simulink model "Wind_turbin."  (R2022b)
settings: Solver=ode45  StartTime=0.0  StopTime=Tsim  FixedStep=5e-5  RelTol=1e-6  EnableMultiTasking=on
values from neighbouring files (symbols this model uses):
  c1 = 0.44    [wind_code.m]
  c2 = 125    [wind_code.m]
  c3 = 0    [wind_code.m]
  c4 = 0    [wind_code.m]
  c5 = 0    [wind_code.m]
  c6 = 6.94    [wind_code.m]
  c7 = 16.5    [wind_code.m]
  c8 = 0    [wind_code.m]
  c9 = -0.002    [wind_code.m]
  N = 80    [wind_code.m]
  p = 2    [wind_code.m]
undefined symbols (not defined in the file or in its folder): A, Cdc, f_n1, fluxm, Jtot, Kcp, ki_dc, ki_m, ki_P_n1, ki_pll_n1, ki_s_n1, kp_dc, kp_md, kp_mq, kp_P_n1, kp_pll_n1, kp_s_n1, Lc_n1, Ld, Lg_n1, Lq, magnitud_delay, pitch, Q_set, Rc_n1, Rg_n1, rho, Rs, Rt, t_step_Q, Vdcref_n1, Vpeak_n1, w_n1
libraries: spsControlledVoltageSourceLib x9, slpidlib x8, spsSeriesRLCBranchLib x7, spsCurrentMeasurementLib x3, spsGroundLib x2, spsThreePhaseVIMeasurementLib x2, spsControlledCurrentSourceLib x2, spsPower3phInstantaneousLib x2, spsPermanentMagnetSynchronousMachineLib x1, spsVoltageMeasurementLib x1, sps_lib x1
(part 2 of 2)

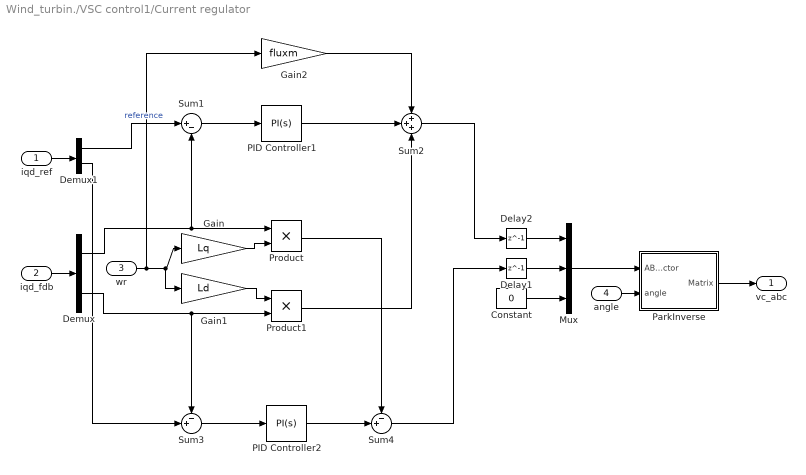
== system Wind_turbin./VSC control1/Current regulator ==
  iqd_ref : Inport
  iqd_fdb : Inport  Port=2
  wr : Inport  Port=3
  angle : Inport  Port=4
  Constant : Constant  Value=0
  Delay1 : Delay  DelayLength=1  InitialCondition=0  SampleTime=magnitud_delay
  Delay2 : Delay  DelayLength=1  InitialCondition=Vpeak_n1  SampleTime=magnitud_delay
  Demux : Demux  Outputs=2
  Demux1 : Demux  Outputs=2
  Gain : Gain  Gain=Lq
  Gain1 : Gain  Gain=Ld
  Gain2 : Gain  Gain=fluxm
  Mux : Mux  Inputs=3
  PID Controller1 : slpidlib/PID Controller  Controller=PI  Form=Parallel  TimeDomain=Continuous-time  UseExternalTs=off  SampleTime=-1  IntegratorMethod=Forward Euler  FilterMethod=Forward Euler  ControllerParametersSource=internal  P=kp_mq  I=ki_m  UseKiTs=off  D=0  N=100  UseFilter=on  TunerSelectOption=Transfer Function Based (PID Tuner App)  InitialConditionSource=internal  InitialConditionForIntegrator=0  InitialConditionForFilter=0  DifferentiatorICPrevScaledInput=0  ExternalReset=none  TrackingMode=off  Kt=1  LimitOutput=off  SatLimitsSource=internal  UpperSaturationLimit=inf  LowerSaturationLimit=-inf  LinearizeAsGain=on  AntiWindupMode=none  Kb=1  LimitIntegrator=off  UpperIntegratorSaturationLimit=inf  LowerIntegratorSaturationLimit=-inf  POutMin=[]  POutMax=[]  IOutMin=[]  IOutMax=[]  DOutMin=[]  DOutMax=[]  NOutMin=[]  NOutMax=[]  SumOutMin=[]  SumOutMax=[]  SaturationOutMin=[]  SaturationOutMax=[]  PParamMin=[]  PParamMax=[]  IParamMin=[]  IParamMax=[]  DParamMin=[]  DParamMax=[]  NParamMin=[]  NParamMax=[]  KbParamMin=[]  KbParamMax=[]  KtParamMin=[]  KtParamMax=[]  KbOutMin=[]  KbOutMax=[]  KtOutMin=[]  KtOutMax=[]  IntegratorOutMin=[]  IntegratorOutMax=[]  FilterOutMin=[]  FilterOutMax=[]  SumI1OutMin=[]  SumI1OutMax=[]  SumI2OutMin=[]  SumI2OutMax=[]  SumI3OutMin=[]  SumI3OutMax=[]  SumI4OutMin=[]  SumI4OutMax=[]  SumDOutMin=[]  SumDOutMax=[]  DifferentiatorOutMin=[]  DifferentiatorOutMax=[]  FilterDiffOutCoefMin=[]  FilterDiffOutCoefMax=[]  ReciprocalOutMin=[]  ReciprocalOutMax=[]  SumDenOutMin=[]  SumDenOutMax=[]  SumNumOutMin=[]  SumNumOutMax=[]  DivideOutMin=[]  DivideOutMax=[]  UdiffTsProdOutMin=[]  UdiffTsProdOutMax=[]  NTsProdOutMin=[]  NTsProdOutMax=[]  UintegralTsProdOutMin=[]  UintegralTsProdOutMax=[]  UngainTsProdOutMin=[]  UngainTsProdOutMax=[]  ClampingZeroOutDataTypeStr=Inherit: Inherit via back propagation  ClampingZeroOutMin=[]  ClampingZeroOutMax=[]  FilterDenConstantOutDataTypeStr=Inherit: Inherit via back propagation  FilterDenConstantOutMin=[]  FilterDenConstantOutMax=[]  PCopyOutDataTypeStr=Inherit: Inherit via back propagation  PCopyOutMin=[]  PCopyOutMax=[]  NCopyOutDataTypeStr=Inherit: Inherit via back propagation  NCopyOutMin=[]  NCopyOutMax=[]  IntegratorContinuousStateAttributes=''  IntegratorStateMustResolveToSignalObject=off  IntegratorRTWStateStorageClass=Auto  FilterContinuousStateAttributes=''  FilterStateMustResolveToSignalObject=off  FilterRTWStateStorageClass=Auto  ParallelPVariant=InternalParameters  IdealPVariant=Disabled  IVariant=InternalParameters  DVariant=Disabled  IntegratorVariant=Continuous  SatVariant=Disabled  AWVariant=Passthrough  PCopyVariant=Disabled  TRVariant=Disabled  FdbkBlocksVariant=Forward  IdealPFdbkVariant=Disabled  SatFdbkVariant=Disabled  DerivativeFilterVariant=Disabled  NVariant=Disabled  NCopyVariant=Disabled_SignalSpec  FilterICVariant=Disabled  IntegratorICVariant=InternalICs  ExternalResetVariant=Disabled  TRSumVariant=Passthrough  SumFdbkVariant=Disabled  SumVariant=Sum_PI  TsampFilterVariant=InternalTs  TsampNgainVariant=Passthrough  TsampIntegralVariant=Passthrough  ExternalSaturationOutDataTypeStr=Inherit: Same as second input
  PID Controller2 : slpidlib/PID Controller  Controller=PI  Form=Parallel  TimeDomain=Continuous-time  UseExternalTs=off  SampleTime=-1  IntegratorMethod=Forward Euler  FilterMethod=Forward Euler  ControllerParametersSource=internal  P=kp_md  I=ki_m  UseKiTs=off  D=0  N=100  UseFilter=on  TunerSelectOption=Transfer Function Based (PID Tuner App)  InitialConditionSource=internal  InitialConditionForIntegrator=0  InitialConditionForFilter=0  DifferentiatorICPrevScaledInput=0  ExternalReset=none  TrackingMode=off  Kt=1  LimitOutput=off  SatLimitsSource=internal  UpperSaturationLimit=inf  LowerSaturationLimit=-inf  LinearizeAsGain=on  AntiWindupMode=none  Kb=1  LimitIntegrator=off  UpperIntegratorSaturationLimit=inf  LowerIntegratorSaturationLimit=-inf  POutMin=[]  POutMax=[]  IOutMin=[]  IOutMax=[]  DOutMin=[]  DOutMax=[]  NOutMin=[]  NOutMax=[]  SumOutMin=[]  SumOutMax=[]  SaturationOutMin=[]  SaturationOutMax=[]  PParamMin=[]  PParamMax=[]  IParamMin=[]  IParamMax=[]  DParamMin=[]  DParamMax=[]  NParamMin=[]  NParamMax=[]  KbParamMin=[]  KbParamMax=[]  KtParamMin=[]  KtParamMax=[]  KbOutMin=[]  KbOutMax=[]  KtOutMin=[]  KtOutMax=[]  IntegratorOutMin=[]  IntegratorOutMax=[]  FilterOutMin=[]  FilterOutMax=[]  SumI1OutMin=[]  SumI1OutMax=[]  SumI2OutMin=[]  SumI2OutMax=[]  SumI3OutMin=[]  SumI3OutMax=[]  SumI4OutMin=[]  SumI4OutMax=[]  SumDOutMin=[]  SumDOutMax=[]  DifferentiatorOutMin=[]  DifferentiatorOutMax=[]  FilterDiffOutCoefMin=[]  FilterDiffOutCoefMax=[]  ReciprocalOutMin=[]  ReciprocalOutMax=[]  SumDenOutMin=[]  SumDenOutMax=[]  SumNumOutMin=[]  SumNumOutMax=[]  DivideOutMin=[]  DivideOutMax=[]  UdiffTsProdOutMin=[]  UdiffTsProdOutMax=[]  NTsProdOutMin=[]  NTsProdOutMax=[]  UintegralTsProdOutMin=[]  UintegralTsProdOutMax=[]  UngainTsProdOutMin=[]  UngainTsProdOutMax=[]  ClampingZeroOutDataTypeStr=Inherit: Inherit via back propagation  ClampingZeroOutMin=[]  ClampingZeroOutMax=[]  FilterDenConstantOutDataTypeStr=Inherit: Inherit via back propagation  FilterDenConstantOutMin=[]  FilterDenConstantOutMax=[]  PCopyOutDataTypeStr=Inherit: Inherit via back propagation  PCopyOutMin=[]  PCopyOutMax=[]  NCopyOutDataTypeStr=Inherit: Inherit via back propagation  NCopyOutMin=[]  NCopyOutMax=[]  IntegratorContinuousStateAttributes=''  IntegratorStateMustResolveToSignalObject=off  IntegratorRTWStateStorageClass=Auto  FilterContinuousStateAttributes=''  FilterStateMustResolveToSignalObject=off  FilterRTWStateStorageClass=Auto  ParallelPVariant=InternalParameters  IdealPVariant=Disabled  IVariant=InternalParameters  DVariant=Disabled  IntegratorVariant=Continuous  SatVariant=Disabled  AWVariant=Passthrough  PCopyVariant=Disabled  TRVariant=Disabled  FdbkBlocksVariant=Forward  IdealPFdbkVariant=Disabled  SatFdbkVariant=Disabled  DerivativeFilterVariant=Disabled  NVariant=Disabled  NCopyVariant=Disabled_SignalSpec  FilterICVariant=Disabled  IntegratorICVariant=InternalICs  ExternalResetVariant=Disabled  TRSumVariant=Passthrough  SumFdbkVariant=Disabled  SumVariant=Sum_PI  TsampFilterVariant=InternalTs  TsampNgainVariant=Passthrough  TsampIntegralVariant=Passthrough  ExternalSaturationOutDataTypeStr=Inherit: Same as second input
  ParkInverse : Subsystem  mask(Gerard){}
      mask help:
      | This block applies the park inverse transfomation from a desired vector.
      | The input Xqd0 refers to the vector in the qd0 frame, and the second input is the angle used in the inverse transformation.
      | The output is the vector in the ABC frame.
      mask Display:
      | port_label('output',1,'Xabc')
      | port_label('input',1,'Xqd0')
      | port_label('input',2,'angle')
  Product : Product  RndMeth=Zero
  Product1 : Product  RndMeth=Zero
  Sum1 : Sum  Inputs=|+-
  Sum2 : Sum  Inputs=+++
  Sum3 : Sum  Inputs=-+|
  Sum4 : Sum  Inputs=-+|
  vc_abc : Outport
  wires:
  iqd_fdb/1 -> Demux/1
  wr/1 -> Gain2/1, Gain1/1, Gain/1
  PID Controller1/1 -> Sum2/2
  Demux/1 -> Sum1/2, Product/1
  Demux/2 -> Product1/2, Sum3/1
  Product1/1 -> Sum2/3
  Product/1 -> Sum4/1
  Constant/1 -> Mux/3
  ParkInverse/1(Matrix) -> vc_abc/1
  iqd_ref/1 -> Demux1/1
  Mux/1 -> ParkInverse/1(ABC vector)
  angle/1 -> ParkInverse/2(angle)
  Sum1/1 -> PID Controller1/1
  Sum3/1 -> PID Controller2/1
  PID Controller2/1 -> Sum4/2
  Demux1/2 -> Sum3/2
  Demux1/1 -> Sum1/1  "reference"
  Sum4/1 -> Delay1/1
  Sum2/1 -> Delay2/1
  Delay1/1 -> Mux/2
  Delay2/1 -> Mux/1
  Gain/1 -> Product/2
  Gain1/1 -> Product1/1
  Gain2/1 -> Sum2/1

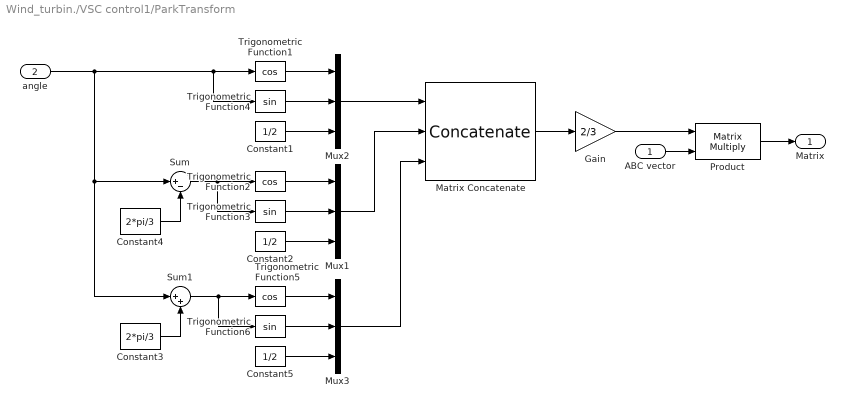
== system Wind_turbin./VSC control1/ParkTransform ==
  ABC vector : Inport
  angle : Inport  Port=2
  Constant1 : Constant  Value=1/2
  Constant2 : Constant  Value=1/2
  Constant3 : Constant  Value=2*pi/3
  Constant4 : Constant  Value=2*pi/3
  Constant5 : Constant  Value=1/2
  Gain : Gain  Gain=2/3
  Matrix Concatenate : Concatenate  NumInputs=3  Mode=Multidimensional array  ConcatenateDimension=2
  Mux1 : Mux  Inputs=3
  Mux2 : Mux  Inputs=3
  Mux3 : Mux  Inputs=3
  Product : Product  Multiplication=Matrix(*)  RndMeth=Zero
  Sum : Sum  Inputs=|+-
  Sum1 : Sum  Inputs=|++
  Trigonometric Function1 : Trigonometry  Operator=cos
  Trigonometric Function2 : Trigonometry  Operator=cos
  Trigonometric Function3 : Trigonometry
  Trigonometric Function4 : Trigonometry
  Trigonometric Function5 : Trigonometry  Operator=cos
  Trigonometric Function6 : Trigonometry
  Matrix : Outport
  wires:
  Matrix Concatenate/1 -> Gain/1
  ABC vector/1 -> Product/2
  Product/1 -> Matrix/1
  Gain/1 -> Product/1
  Constant4/1 -> Sum/2
  Constant3/1 -> Sum1/2
  angle/1 -> Trigonometric Function4/1, Trigonometric Function1/1, Sum1/1, Sum/1
  Trigonometric Function3/1 -> Mux1/2
  Trigonometric Function2/1 -> Mux1/1
  Constant2/1 -> Mux1/3
  Sum/1 -> Trigonometric Function3/1, Trigonometric Function2/1
  Trigonometric Function4/1 -> Mux2/2
  Trigonometric Function1/1 -> Mux2/1
  Constant1/1 -> Mux2/3
  Trigonometric Function6/1 -> Mux3/2
  Trigonometric Function5/1 -> Mux3/1
  Constant5/1 -> Mux3/3
  Sum1/1 -> Trigonometric Function6/1, Trigonometric Function5/1
  Mux1/1 -> Matrix Concatenate/2
  Mux2/1 -> Matrix Concatenate/1
  Mux3/1 -> Matrix Concatenate/3

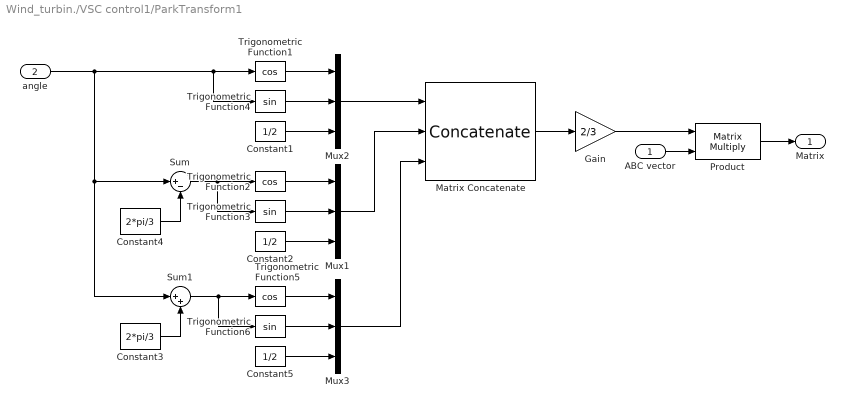
== system Wind_turbin./VSC control1/ParkTransform1 ==
  ABC vector : Inport
  angle : Inport  Port=2
  Constant1 : Constant  Value=1/2
  Constant2 : Constant  Value=1/2
  Constant3 : Constant  Value=2*pi/3
  Constant4 : Constant  Value=2*pi/3
  Constant5 : Constant  Value=1/2
  Gain : Gain  Gain=2/3
  Matrix Concatenate : Concatenate  NumInputs=3  Mode=Multidimensional array  ConcatenateDimension=2
  Mux1 : Mux  Inputs=3
  Mux2 : Mux  Inputs=3
  Mux3 : Mux  Inputs=3
  Product : Product  Multiplication=Matrix(*)  RndMeth=Zero
  Sum : Sum  Inputs=|+-
  Sum1 : Sum  Inputs=|++
  Trigonometric Function1 : Trigonometry  Operator=cos
  Trigonometric Function2 : Trigonometry  Operator=cos
  Trigonometric Function3 : Trigonometry
  Trigonometric Function4 : Trigonometry
  Trigonometric Function5 : Trigonometry  Operator=cos
  Trigonometric Function6 : Trigonometry
  Matrix : Outport
  wires:
  Matrix Concatenate/1 -> Gain/1
  ABC vector/1 -> Product/2
  Product/1 -> Matrix/1
  Gain/1 -> Product/1
  Constant4/1 -> Sum/2
  Constant3/1 -> Sum1/2
  angle/1 -> Trigonometric Function4/1, Trigonometric Function1/1, Sum1/1, Sum/1
  Trigonometric Function3/1 -> Mux1/2
  Trigonometric Function2/1 -> Mux1/1
  Constant2/1 -> Mux1/3
  Sum/1 -> Trigonometric Function3/1, Trigonometric Function2/1
  Trigonometric Function4/1 -> Mux2/2
  Trigonometric Function1/1 -> Mux2/1
  Constant1/1 -> Mux2/3
  Trigonometric Function6/1 -> Mux3/2
  Trigonometric Function5/1 -> Mux3/1
  Constant5/1 -> Mux3/3
  Sum1/1 -> Trigonometric Function6/1, Trigonometric Function5/1
  Mux1/1 -> Matrix Concatenate/2
  Mux2/1 -> Matrix Concatenate/1
  Mux3/1 -> Matrix Concatenate/3

== system Wind_turbin./VSC control1/Q loop ==
  Q_ref : Inport
  Q : Inport  Port=2
  Gain2 : Gain  Gain=2/(3*Vpeak_n1)
  PID Controller : slpidlib/PID Controller  Controller=PI  Form=Parallel  TimeDomain=Continuous-time  UseExternalTs=off  SampleTime=-1  IntegratorMethod=Forward Euler  FilterMethod=Forward Euler  ControllerParametersSource=internal  P=kp_P_n1  I=ki_P_n1  UseKiTs=off  D=0  N=100  UseFilter=on  TunerSelectOption=Transfer Function Based (PID Tuner App)  InitialConditionSource=internal  InitialConditionForIntegrator=0  InitialConditionForFilter=0  DifferentiatorICPrevScaledInput=0  ExternalReset=none  TrackingMode=off  Kt=1  LimitOutput=off  SatLimitsSource=internal  UpperSaturationLimit=inf  LowerSaturationLimit=-inf  LinearizeAsGain=on  AntiWindupMode=none  Kb=1  LimitIntegrator=off  UpperIntegratorSaturationLimit=inf  LowerIntegratorSaturationLimit=-inf  POutMin=[]  POutMax=[]  IOutMin=[]  IOutMax=[]  DOutMin=[]  DOutMax=[]  NOutMin=[]  NOutMax=[]  SumOutMin=[]  SumOutMax=[]  SaturationOutMin=[]  SaturationOutMax=[]  PParamMin=[]  PParamMax=[]  IParamMin=[]  IParamMax=[]  DParamMin=[]  DParamMax=[]  NParamMin=[]  NParamMax=[]  KbParamMin=[]  KbParamMax=[]  KtParamMin=[]  KtParamMax=[]  KbOutMin=[]  KbOutMax=[]  KtOutMin=[]  KtOutMax=[]  IntegratorOutMin=[]  IntegratorOutMax=[]  FilterOutMin=[]  FilterOutMax=[]  SumI1OutMin=[]  SumI1OutMax=[]  SumI2OutMin=[]  SumI2OutMax=[]  SumI3OutMin=[]  SumI3OutMax=[]  SumI4OutMin=[]  SumI4OutMax=[]  SumDOutMin=[]  SumDOutMax=[]  DifferentiatorOutMin=[]  DifferentiatorOutMax=[]  FilterDiffOutCoefMin=[]  FilterDiffOutCoefMax=[]  ReciprocalOutMin=[]  ReciprocalOutMax=[]  SumDenOutMin=[]  SumDenOutMax=[]  SumNumOutMin=[]  SumNumOutMax=[]  DivideOutMin=[]  DivideOutMax=[]  UdiffTsProdOutMin=[]  UdiffTsProdOutMax=[]  NTsProdOutMin=[]  NTsProdOutMax=[]  UintegralTsProdOutMin=[]  UintegralTsProdOutMax=[]  UngainTsProdOutMin=[]  UngainTsProdOutMax=[]  ClampingZeroOutDataTypeStr=Inherit: Inherit via back propagation  ClampingZeroOutMin=[]  ClampingZeroOutMax=[]  FilterDenConstantOutDataTypeStr=Inherit: Inherit via back propagation  FilterDenConstantOutMin=[]  FilterDenConstantOutMax=[]  PCopyOutDataTypeStr=Inherit: Inherit via back propagation  PCopyOutMin=[]  PCopyOutMax=[]  NCopyOutDataTypeStr=Inherit: Inherit via back propagation  NCopyOutMin=[]  NCopyOutMax=[]  IntegratorContinuousStateAttributes=''  IntegratorStateMustResolveToSignalObject=off  IntegratorRTWStateStorageClass=Auto  FilterContinuousStateAttributes=''  FilterStateMustResolveToSignalObject=off  FilterRTWStateStorageClass=Auto  ParallelPVariant=InternalParameters  IdealPVariant=Disabled  IVariant=InternalParameters  DVariant=Disabled  IntegratorVariant=Continuous  SatVariant=Disabled  AWVariant=Passthrough  PCopyVariant=Disabled  TRVariant=Disabled  FdbkBlocksVariant=Forward  IdealPFdbkVariant=Disabled  SatFdbkVariant=Disabled  DerivativeFilterVariant=Disabled  NVariant=Disabled  NCopyVariant=Disabled_SignalSpec  FilterICVariant=Disabled  IntegratorICVariant=InternalICs  ExternalResetVariant=Disabled  TRSumVariant=Passthrough  SumFdbkVariant=Disabled  SumVariant=Sum_PI  TsampFilterVariant=InternalTs  TsampNgainVariant=Passthrough  TsampIntegralVariant=Passthrough  ExternalSaturationOutDataTypeStr=Inherit: Same as second input
  Scope3 : Scope
  Sum1 : Sum  Inputs=|+-
  is_d_ref : Outport
  wires:
  PID Controller/1 -> Gain2/1
  Q_ref/1 -> Sum1/1
  Sum1/1 -> Scope3/1, PID Controller/1
  Q/1 -> Sum1/2
  Gain2/1 -> is_d_ref/1

== system Wind_turbin./Wind Turbine Power/Cp ==
  In1 : Inport
  pitch angle : Inport  Port=2
  Add : Sum  Inputs=+---
  Constant1 : Constant  Value=c6
  Constant3 : Constant  Value=c5
  Gain : Gain  Gain=c3
  Gain1 : Gain  Gain=c4
  Gain2 : Gain  Gain=c2
  Gain3 : Gain  Gain=c1
  Gain4 : Gain  Gain=-c7
  Math Function : Math
  Math Function2 : Math  Operator=pow
  Product2 : Product
  Cp : Outport
  wires:
  Gain2/1 -> Add/1
  Constant1/1 -> Add/2
  In1/1 -> Gain2/1, Gain4/1
  Gain4/1 -> Math Function/1
  Product2/1 -> Gain3/1
  Gain3/1 -> Cp/1
  pitch angle/1 -> Gain/1, Math Function2/1
  Constant3/1 -> Math Function2/2
  Math Function2/1 -> Gain1/1
  Gain/1 -> Add/3
  Gain1/1 -> Add/4
  Math Function/1 -> Product2/1
  Add/1 -> Product2/2

== system Wind_turbin./Wind Turbine Power/alfa ==
  tip speed : Inport
  pitch angle : Inport  Port=2
  Add1 : Sum
  Add2 : Sum
  Add3 : Sum  Inputs=+-
  Constant : Constant
  Constant1 : Constant  Value=c9
  Divide : Product  Inputs=*/
  Gain : Gain  Gain=c8
  Math Function : Math  Operator=reciprocal
  Product : Product  Inputs=3
  Out1 : Outport
  wires:
  Add3/1 -> Out1/1
  Math Function/1 -> Add3/1
  pitch angle/1 -> Product/1, Product/3, Product/2, Gain/1
  Add1/1 -> Math Function/1
  tip speed/1 -> Add1/1
  Gain/1 -> Add1/2
  Product/1 -> Add2/1
  Constant/1 -> Add2/2
  Add2/1 -> Divide/2
  Constant1/1 -> Divide/1
  Divide/1 -> Add3/2

== system Wind_turbin./VSC control/Current regulator/ParkInverse ==
  ABC vector : Inport
  angle : Inport  Port=2
  Constant4 : Constant  Value=2*pi/3
  Constant5 : Constant  Value=2*pi/3
  Constant9 : Constant
  Matrix Concatenate2 : Concatenate  NumInputs=3  Mode=Multidimensional array  ConcatenateDimension=2
  Mux6 : Mux  Inputs=3
  Mux7 : Mux  Inputs=3
  Product : Product  Multiplication=Matrix(*)  RndMeth=Zero
  Sum : Sum  Inputs=|+-
  Sum1 : Sum  Inputs=|++
  Trigonometric Function8 : Trigonometry  Operator=cos
  Trigonometric Function9 : Trigonometry
  Matrix : Outport
  wires:
  angle/1 -> Sum1/1, Sum/1, Mux6/1
  Constant5/1 -> Sum1/2
  Constant4/1 -> Sum/2
  Product/1 -> Matrix/1
  ABC vector/1 -> Product/2
  Sum/1 -> Mux6/2
  Sum1/1 -> Mux6/3
  Constant9/1 -> Mux7/3, Mux7/1, Mux7/2
  Trigonometric Function8/1 -> Matrix Concatenate2/1
  Trigonometric Function9/1 -> Matrix Concatenate2/2
  Mux6/1 -> Trigonometric Function9/1, Trigonometric Function8/1
  Mux7/1 -> Matrix Concatenate2/3
  Matrix Concatenate2/1 -> Product/1

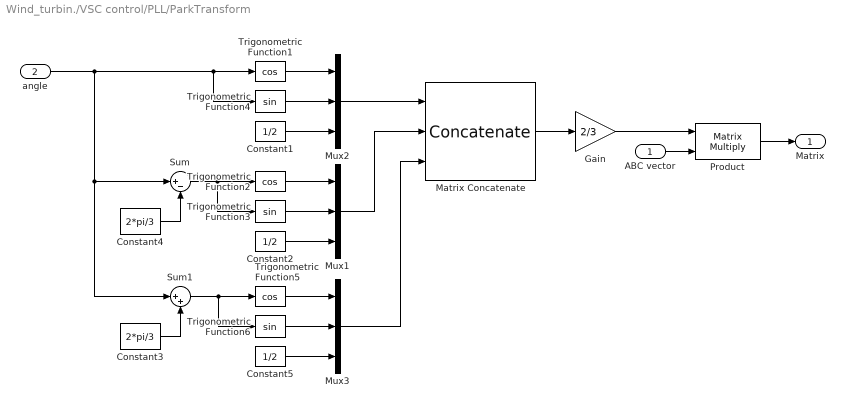
== system Wind_turbin./VSC control/PLL/ParkTransform ==
  ABC vector : Inport
  angle : Inport  Port=2
  Constant1 : Constant  Value=1/2
  Constant2 : Constant  Value=1/2
  Constant3 : Constant  Value=2*pi/3
  Constant4 : Constant  Value=2*pi/3
  Constant5 : Constant  Value=1/2
  Gain : Gain  Gain=2/3
  Matrix Concatenate : Concatenate  NumInputs=3  Mode=Multidimensional array  ConcatenateDimension=2
  Mux1 : Mux  Inputs=3
  Mux2 : Mux  Inputs=3
  Mux3 : Mux  Inputs=3
  Product : Product  Multiplication=Matrix(*)  RndMeth=Zero
  Sum : Sum  Inputs=|+-
  Sum1 : Sum  Inputs=|++
  Trigonometric Function1 : Trigonometry  Operator=cos
  Trigonometric Function2 : Trigonometry  Operator=cos
  Trigonometric Function3 : Trigonometry
  Trigonometric Function4 : Trigonometry
  Trigonometric Function5 : Trigonometry  Operator=cos
  Trigonometric Function6 : Trigonometry
  Matrix : Outport
  wires:
  Matrix Concatenate/1 -> Gain/1
  ABC vector/1 -> Product/2
  Product/1 -> Matrix/1
  Gain/1 -> Product/1
  Constant4/1 -> Sum/2
  Constant3/1 -> Sum1/2
  angle/1 -> Trigonometric Function4/1, Trigonometric Function1/1, Sum1/1, Sum/1
  Trigonometric Function3/1 -> Mux1/2
  Trigonometric Function2/1 -> Mux1/1
  Constant2/1 -> Mux1/3
  Sum/1 -> Trigonometric Function3/1, Trigonometric Function2/1
  Trigonometric Function4/1 -> Mux2/2
  Trigonometric Function1/1 -> Mux2/1
  Constant1/1 -> Mux2/3
  Trigonometric Function6/1 -> Mux3/2
  Trigonometric Function5/1 -> Mux3/1
  Constant5/1 -> Mux3/3
  Sum1/1 -> Trigonometric Function6/1, Trigonometric Function5/1
  Mux1/1 -> Matrix Concatenate/2
  Mux2/1 -> Matrix Concatenate/1
  Mux3/1 -> Matrix Concatenate/3

== system Wind_turbin./VSC control1/Current regulator/ParkInverse ==
  ABC vector : Inport
  angle : Inport  Port=2
  Constant4 : Constant  Value=2*pi/3
  Constant5 : Constant  Value=2*pi/3
  Constant9 : Constant
  Matrix Concatenate2 : Concatenate  NumInputs=3  Mode=Multidimensional array  ConcatenateDimension=2
  Mux6 : Mux  Inputs=3
  Mux7 : Mux  Inputs=3
  Product : Product  Multiplication=Matrix(*)  RndMeth=Zero
  Sum : Sum  Inputs=|+-
  Sum1 : Sum  Inputs=|++
  Trigonometric Function8 : Trigonometry  Operator=cos
  Trigonometric Function9 : Trigonometry
  Matrix : Outport
  wires:
  angle/1 -> Sum1/1, Sum/1, Mux6/1
  Constant5/1 -> Sum1/2
  Constant4/1 -> Sum/2
  Product/1 -> Matrix/1
  ABC vector/1 -> Product/2
  Sum/1 -> Mux6/2
  Sum1/1 -> Mux6/3
  Constant9/1 -> Mux7/3, Mux7/1, Mux7/2
  Trigonometric Function8/1 -> Matrix Concatenate2/1
  Trigonometric Function9/1 -> Matrix Concatenate2/2
  Mux6/1 -> Trigonometric Function9/1, Trigonometric Function8/1
  Mux7/1 -> Matrix Concatenate2/3
  Matrix Concatenate2/1 -> Product/1
